simulink model "s_c856m4k_cd"  (R2016b)
(part 2 of 60)

      mask init:
      | pipeline_init(gcb,'latency',latency);
      settings: AttributesFormatString=Latency = %<latency>
      mask Display:
      | port_label('input', 1, 'd');
      | port_label('output', 1, 'q');
      | disp(['Z^-', num2str(latency)]);
  pipeline78 : Subsystem  AncestorBlock=casper_library_delays/pipeline  mask(pipeline){latency=2}
      mask help:
      | An explicitly laid-out delay line to avoid mapping to SRL16s
      | for use in pipelining to help achieve timing closure.
      mask init:
      | pipeline_init(gcb,'latency',latency);
      settings: AttributesFormatString=Latency = %<latency>
      mask Display:
      | port_label('input', 1, 'd');
      | port_label('output', 1, 'q');
      | disp(['Z^-', num2str(latency)]);
  pipeline8 : Subsystem  AncestorBlock=casper_library_delays/pipeline  mask(pipeline){latency=2}
      mask help:
      | An explicitly laid-out delay line to avoid mapping to SRL16s
      | for use in pipelining to help achieve timing closure.
      mask init:
      | pipeline_init(gcb,'latency',latency);
      settings: AttributesFormatString=Latency = %<latency>
      mask Display:
      | port_label('input', 1, 'd');
      | port_label('output', 1, 'q');
      | disp(['Z^-', num2str(latency)]);
  pipeline84 : Subsystem  AncestorBlock=casper_library_delays/pipeline  mask(pipeline){latency=2}
      mask help:
      | An explicitly laid-out delay line to avoid mapping to SRL16s
      | for use in pipelining to help achieve timing closure.
      mask init:
      | pipeline_init(gcb,'latency',latency);
      settings: AttributesFormatString=Latency = %<latency>
      mask Display:
      | port_label('input', 1, 'd');
      | port_label('output', 1, 'q');
      | disp(['Z^-', num2str(latency)]);
  pipeline88 : Subsystem  AncestorBlock=casper_library_delays/pipeline  mask(pipeline){latency=1}
      mask help:
      | An explicitly laid-out delay line to avoid mapping to SRL16s
      | for use in pipelining to help achieve timing closure.
      mask init:
      | pipeline_init(gcb,'latency',latency);
      settings: AttributesFormatString=Latency = %<latency>
      mask Display:
      | port_label('input', 1, 'd');
      | port_label('output', 1, 'q');
      | disp(['Z^-', num2str(latency)]);
  pipeline9 : Subsystem  AncestorBlock=casper_library_delays/pipeline  mask(pipeline){latency=2}
      mask help:
      | An explicitly laid-out delay line to avoid mapping to SRL16s
      | for use in pipelining to help achieve timing closure.
      mask init:
      | pipeline_init(gcb,'latency',latency);
      settings: AttributesFormatString=Latency = %<latency>
      mask Display:
      | port_label('input', 1, 'd');
      | port_label('output', 1, 'q');
      | disp(['Z^-', num2str(latency)]);
  pipeline96 : Subsystem  AncestorBlock=casper_library_delays/pipeline  mask(pipeline){latency=2}
      mask help:
      | An explicitly laid-out delay line to avoid mapping to SRL16s
      | for use in pipelining to help achieve timing closure.
      mask init:
      | pipeline_init(gcb,'latency',latency);
      settings: AttributesFormatString=Latency = %<latency>
      mask Display:
      | port_label('input', 1, 'd');
      | port_label('output', 1, 'q');
      | disp(['Z^-', num2str(latency)]);
  pipeline97 : Subsystem  AncestorBlock=casper_library_delays/pipeline  mask(pipeline){latency=2}
      mask help:
      | An explicitly laid-out delay line to avoid mapping to SRL16s
      | for use in pipelining to help achieve timing closure.
      mask init:
      | pipeline_init(gcb,'latency',latency);
      settings: AttributesFormatString=Latency = %<latency>
      mask Display:
      | port_label('input', 1, 'd');
      | port_label('output', 1, 'q');
      | disp(['Z^-', num2str(latency)]);
  pipeline98 : Subsystem  AncestorBlock=casper_library_delays/pipeline  mask(pipeline){latency=2}
      mask help:
      | An explicitly laid-out delay line to avoid mapping to SRL16s
      | for use in pipelining to help achieve timing closure.
      mask init:
      | pipeline_init(gcb,'latency',latency);
      settings: AttributesFormatString=Latency = %<latency>
      mask Display:
      | port_label('input', 1, 'd');
      | port_label('output', 1, 'q');
      | disp(['Z^-', num2str(latency)]);
  pipeline99 : Subsystem  AncestorBlock=casper_library_delays/pipeline  mask(pipeline){latency=2}
      mask help:
      | An explicitly laid-out delay line to avoid mapping to SRL16s
      | for use in pipelining to help achieve timing closure.
      mask init:
      | pipeline_init(gcb,'latency',latency);
      settings: AttributesFormatString=Latency = %<latency>
      mask Display:
      | port_label('input', 1, 'd');
      | port_label('output', 1, 'q');
      | disp(['Z^-', num2str(latency)]);
  pkt_cnt0 : Subsystem
  rx_dest_ip : Subsystem  Tag=xps:sw_reg  AncestorBlock=xps_library/software register  mask(swreg){io_dir=To Processor, io_delay=0, sample_period=1, names=reg, bitwidths=32, bin_pts=0, arith_types=0, sim_port=off, show_format=on}
      mask prompts: io_dir "I/O direction"; io_delay "I/O delay"; sample_period "Sample period"; names "Bitfield names [msb...lsb]"; bitwidths "Bitfield widths"; bin_pts "Bitfield binary pts"; arith_types "Bitfield types, ufix=0, fix=1, bool=2"; sim_port "Provide sim input/output?"; show_format "Print format string?"
      mask help: A 32-bit software-accessible register. Can be divided into bitfields of varying widths and types using the fields in the block mask.
      mask init:
      | swreg_init(gcb)
      settings: AttributesFormatString=1output:uf32.0 = 32 bits
      mask TypeOptions io_dir: To Processor | From Processor
      mask Callback io_dir:
      | mask_enables = get_param(gcb, 'MaskEnables');
      | mask_names = get_param(gcb, 'MaskNames');
      | if strcmp(get_param(gcb, 'io_dir'), 'To Processor'),
      |     mask_enables{ismember(mask_names, 'sample_period')} = 'off';
      | else
      |     mask_enables{ismember(mask_names, 'sample_period')} = 'on';
      | end
      | set_param(gcb, 'MaskEnables', mask_enables);
  rx_dest_port : Subsystem  Tag=xps:sw_reg  AncestorBlock=xps_library/software register  mask(swreg){io_dir=To Processor, io_delay=0, sample_period=1, names=reg, bitwidths=16, bin_pts=0, arith_types=0, sim_port=off, show_format=on}
      mask prompts: io_dir "I/O direction"; io_delay "I/O delay"; sample_period "Sample period"; names "Bitfield names [msb...lsb]"; bitwidths "Bitfield widths"; bin_pts "Bitfield binary pts"; arith_types "Bitfield types, ufix=0, fix=1, bool=2"; sim_port "Provide sim input/output?"; show_format "Print format string?"
      mask help: A 32-bit software-accessible register. Can be divided into bitfields of varying widths and types using the fields in the block mask.
      mask init:
      | swreg_init(gcb)
      settings: AttributesFormatString=1output:uf16.0 = 16 bits
      mask TypeOptions io_dir: To Processor | From Processor
      mask Callback io_dir:
      | mask_enables = get_param(gcb, 'MaskEnables');
      | mask_names = get_param(gcb, 'MaskNames');
      | if strcmp(get_param(gcb, 'io_dir'), 'To Processor'),
      |     mask_enables{ismember(mask_names, 'sample_period')} = 'off';
      | else
      |     mask_enables{ismember(mask_names, 'sample_period')} = 'on';
      | end
      | set_param(gcb, 'MaskEnables', mask_enables);
  rx_integrity_check0 : Subsystem
  rx_pkt_cnt_bad : Subsystem  Tag=xps:sw_reg  AncestorBlock=xps_library/software register  mask(swreg){io_dir=To Processor, io_delay=0, sample_period=1, names=reg, bitwidths=32, bin_pts=0, arith_types=0, sim_port=off, show_format=on}
      mask prompts: io_dir "I/O direction"; io_delay "I/O delay"; sample_period "Sample period"; names "Bitfield names [msb...lsb]"; bitwidths "Bitfield widths"; bin_pts "Bitfield binary pts"; arith_types "Bitfield types, ufix=0, fix=1, bool=2"; sim_port "Provide sim input/output?"; show_format "Print format string?"
      mask help: A 32-bit software-accessible register. Can be divided into bitfields of varying widths and types using the fields in the block mask.
      mask init:
      | swreg_init(gcb)
      settings: AttributesFormatString=1output:uf32.0 = 32 bits
      mask TypeOptions io_dir: To Processor | From Processor
      mask Callback io_dir:
      | mask_enables = get_param(gcb, 'MaskEnables');
      | mask_names = get_param(gcb, 'MaskNames');
      | if strcmp(get_param(gcb, 'io_dir'), 'To Processor'),
      |     mask_enables{ismember(mask_names, 'sample_period')} = 'off';
      | else
      |     mask_enables{ismember(mask_names, 'sample_period')} = 'on';
      | end
      | set_param(gcb, 'MaskEnables', mask_enables);
  rx_pkt_cnt_ok : Subsystem  Tag=xps:sw_reg  AncestorBlock=xps_library/software register  mask(swreg){io_dir=To Processor, io_delay=0, sample_period=1, names=reg, bitwidths=32, bin_pts=0, arith_types=0, sim_port=off, show_format=on}
      mask prompts: io_dir "I/O direction"; io_delay "I/O delay"; sample_period "Sample period"; names "Bitfield names [msb...lsb]"; bitwidths "Bitfield widths"; bin_pts "Bitfield binary pts"; arith_types "Bitfield types, ufix=0, fix=1, bool=2"; sim_port "Provide sim input/output?"; show_format "Print format string?"
      mask help: A 32-bit software-accessible register. Can be divided into bitfields of varying widths and types using the fields in the block mask.
      mask init:
      | swreg_init(gcb)
      settings: AttributesFormatString=1output:uf32.0 = 32 bits
      mask TypeOptions io_dir: To Processor | From Processor
      mask Callback io_dir:
      | mask_enables = get_param(gcb, 'MaskEnables');
      | mask_names = get_param(gcb, 'MaskNames');
      | if strcmp(get_param(gcb, 'io_dir'), 'To Processor'),
      |     mask_enables{ismember(mask_names, 'sample_period')} = 'off';
      | else
      |     mask_enables{ismember(mask_names, 'sample_period')} = 'on';
      | end
      | set_param(gcb, 'MaskEnables', mask_enables);
  rx_src_ip : Subsystem  Tag=xps:sw_reg  AncestorBlock=xps_library/software register  mask(swreg){io_dir=To Processor, io_delay=0, sample_period=1, names=reg, bitwidths=32, bin_pts=0, arith_types=0, sim_port=off, show_format=on}
      mask prompts: io_dir "I/O direction"; io_delay "I/O delay"; sample_period "Sample period"; names "Bitfield names [msb...lsb]"; bitwidths "Bitfield widths"; bin_pts "Bitfield binary pts"; arith_types "Bitfield types, ufix=0, fix=1, bool=2"; sim_port "Provide sim input/output?"; show_format "Print format string?"
      mask help: A 32-bit software-accessible register. Can be divided into bitfields of varying widths and types using the fields in the block mask.
      mask init:
      | swreg_init(gcb)
      settings: AttributesFormatString=1output:uf32.0 = 32 bits
      mask TypeOptions io_dir: To Processor | From Processor
      mask Callback io_dir:
      | mask_enables = get_param(gcb, 'MaskEnables');
      | mask_names = get_param(gcb, 'MaskNames');
      | if strcmp(get_param(gcb, 'io_dir'), 'To Processor'),
      |     mask_enables{ismember(mask_names, 'sample_period')} = 'off';
      | else
      |     mask_enables{ismember(mask_names, 'sample_period')} = 'on';
      | end
      | set_param(gcb, 'MaskEnables', mask_enables);
  rx_src_port : Subsystem  Tag=xps:sw_reg  AncestorBlock=xps_library/software register  mask(swreg){io_dir=To Processor, io_delay=0, sample_period=1, names=reg, bitwidths=16, bin_pts=0, arith_types=0, sim_port=off, show_format=on}
      mask prompts: io_dir "I/O direction"; io_delay "I/O delay"; sample_period "Sample period"; names "Bitfield names [msb...lsb]"; bitwidths "Bitfield widths"; bin_pts "Bitfield binary pts"; arith_types "Bitfield types, ufix=0, fix=1, bool=2"; sim_port "Provide sim input/output?"; show_format "Print format string?"
      mask help: A 32-bit software-accessible register. Can be divided into bitfields of varying widths and types using the fields in the block mask.
      mask init:
      | swreg_init(gcb)
      settings: AttributesFormatString=1output:uf16.0 = 16 bits
      mask TypeOptions io_dir: To Processor | From Processor
      mask Callback io_dir:
      | mask_enables = get_param(gcb, 'MaskEnables');
      | mask_names = get_param(gcb, 'MaskNames');
      | if strcmp(get_param(gcb, 'io_dir'), 'To Processor'),
      |     mask_enables{ismember(mask_names, 'sample_period')} = 'off';
      | else
      |     mask_enables{ismember(mask_names, 'sample_period')} = 'on';
      | end
      | set_param(gcb, 'MaskEnables', mask_enables);
  rx_status : Subsystem  Tag=xps:sw_reg  AncestorBlock=xps_library/software_register  mask(swreg){io_dir=To Processor, io_delay=0, sample_period=1, names=[badframe overrun valid eof], bitwidths=8, bin_pts=0, arith_types=0, sim_port=off, show_format=on}
      mask prompts: io_dir "I/O direction"; io_delay "I/O delay"; sample_period "Sample period"; names "Bitfield names [msb...lsb]"; bitwidths "Bitfield widths"; bin_pts "Bitfield binary pts"; arith_types "Bitfield types, ufix=0, fix=1, bool=2"; sim_port "Provide sim input/output?"; show_format "Print format string?"
      mask help: A 32-bit software-accessible register. Can be divided into bitfields of varying widths and types using the fields in the block mask.
      mask init:
      | swreg_init(gcb)
      settings: AttributesFormatString=4 outputs:uf8.0,uf8.0,uf8.0,uf8.0 = 32 bits
      mask TypeOptions io_dir: To Processor | From Processor
      mask Callback io_dir:
      | mask_enables = get_param(gcb, 'MaskEnables');
      | mask_names = get_param(gcb, 'MaskNames');
      | if strcmp(get_param(gcb, 'io_dir'), 'To Processor'),
      |     mask_enables{ismember(mask_names, 'sample_period')} = 'off';
      | else
      |     mask_enables{ismember(mask_names, 'sample_period')} = 'on';
      | end
      | set_param(gcb, 'MaskEnables', mask_enables);
      mask DialogControl ParameterTabVar0 Prompt: Setup
  rx_wrd_cnt_bad : Subsystem  Tag=xps:sw_reg  AncestorBlock=xps_library/software register  mask(swreg){io_dir=To Processor, io_delay=0, sample_period=1, names=reg, bitwidths=32, bin_pts=0, arith_types=0, sim_port=off, show_format=on}
      mask prompts: io_dir "I/O direction"; io_delay "I/O delay"; sample_period "Sample period"; names "Bitfield names [msb...lsb]"; bitwidths "Bitfield widths"; bin_pts "Bitfield binary pts"; arith_types "Bitfield types, ufix=0, fix=1, bool=2"; sim_port "Provide sim input/output?"; show_format "Print format string?"
      mask help: A 32-bit software-accessible register. Can be divided into bitfields of varying widths and types using the fields in the block mask.
      mask init:
      | swreg_init(gcb)
      settings: AttributesFormatString=1output:uf32.0 = 32 bits
      mask TypeOptions io_dir: To Processor | From Processor
      mask Callback io_dir:
      | mask_enables = get_param(gcb, 'MaskEnables');
      | mask_names = get_param(gcb, 'MaskNames');
      | if strcmp(get_param(gcb, 'io_dir'), 'To Processor'),
      |     mask_enables{ismember(mask_names, 'sample_period')} = 'off';
      | else
      |     mask_enables{ismember(mask_names, 'sample_period')} = 'on';
      | end
      | set_param(gcb, 'MaskEnables', mask_enables);
  rx_wrd_cnt_missing : Subsystem  Tag=xps:sw_reg  AncestorBlock=xps_library/software register  mask(swreg){io_dir=To Processor, io_delay=0, sample_period=1, names=reg, bitwidths=32, bin_pts=0, arith_types=0, sim_port=off, show_format=on}
      mask prompts: io_dir "I/O direction"; io_delay "I/O delay"; sample_period "Sample period"; names "Bitfield names [msb...lsb]"; bitwidths "Bitfield widths"; bin_pts "Bitfield binary pts"; arith_types "Bitfield types, ufix=0, fix=1, bool=2"; sim_port "Provide sim input/output?"; show_format "Print format string?"
      mask help: A 32-bit software-accessible register. Can be divided into bitfields of varying widths and types using the fields in the block mask.
      mask init:
      | swreg_init(gcb)
      settings: AttributesFormatString=1output:uf32.0 = 32 bits
      mask TypeOptions io_dir: To Processor | From Processor
      mask Callback io_dir:
      | mask_enables = get_param(gcb, 'MaskEnables');
      | mask_names = get_param(gcb, 'MaskNames');
      | if strcmp(get_param(gcb, 'io_dir'), 'To Processor'),
      |     mask_enables{ismember(mask_names, 'sample_period')} = 'off';
      | else
      |     mask_enables{ismember(mask_names, 'sample_period')} = 'on';
      | end
      | set_param(gcb, 'MaskEnables', mask_enables);
  snap_adc0 : Subsystem  Tag=casper:bitsnap  AncestorBlock=casper_library_scopes/bitfield snapshot  mask(bitsnap){io_names=[d0 d1 d2 d3 d4 d5 d6 d7 p1_d0 p1_d1 p1_d2 p1_d3 p1_d4_u8], io_widths=[10 10 10 10 10 10 10 10 10 10 10 10 8], io_bps=[9 9 9 9 9 9 9 9 9 9 9 9 0], io_types=[1 1 1 1 1 1 1 1 1 1 1 1 0], snap_storage=bram, snap_dram_dimm=2, snap_dram_clock=250, snap_nsamples=11, snap_data_width=128, snap_offset=on, snap_circap=off, snap_value=off, snap_use_dsp48=off, snap_delay=0, extra_names=[c d], extra_widths=[30 2], extra_bps=[0 0], extra_types=[0 0]}
      mask prompts: io_names "Names [msb...lsb]"; io_widths "Widths [msb...lsb]"; io_bps "Binary pts [msb...lsb]"; io_types "Data types [msb...lsb], ufix=0, fix=1, bool=2"; snap_storage "Storage medium"; snap_dram_dimm "DRAM dimm"; snap_dram_clock "DRAM clock rate"; snap_nsamples "Number of Samples (2^?)"; snap_data_width "Data width"; snap_offset "Start delay support"; snap_circap "Circular capture support"; snap_value "Extra value capture support"; snap_use_dsp48 "Use DSP48s to implement counters"; snap_delay "Pre-snapshot delay"; extra_names "Names [msb...lsb]"; extra_widths "Widths [msb...lsb]"; extra_bps "Binary pts [msb...lsb]"; extra_types "Data types [msb...lsb], ufix=0, fix=1, bool=2"
      mask help:
      | A wrapped snapshot block. Allows specification of inputs to a snapblock word so the toolflow can automatically set up the scope.
      | See documentation for snapshot for explanation of parameters.
      mask init:
      | bitsnap_init(gcb);
      mask TypeOptions snap_storage: bram | dram
      mask Callback snap_storage: bitsnap_callback();
      mask TypeOptions snap_dram_dimm: 1 | 2 | 3 | 4
      mask TypeOptions snap_dram_clock: 200 | 250 | 266 | 300 | 333
      mask TypeOptions snap_data_width: 8 | 16 | 32 | 64 | 128
      mask Callback snap_value: bitsnap_callback();
  snap_adc1 : Subsystem  Tag=casper:bitsnap  AncestorBlock=casper_library_scopes/bitfield snapshot  mask(bitsnap){io_names=[p1_d4_l2 p1_d5 p1_d6 p1_d7], io_widths=[2 10 10 10], io_bps=[0 9 9 9], io_types=[0 1 1 1], snap_storage=bram, snap_dram_dimm=2, snap_dram_clock=250, snap_nsamples=11, snap_data_width=32, snap_offset=on, snap_circap=off, snap_value=off, snap_use_dsp48=off, snap_delay=0, extra_names=[c d], extra_widths=[30 2], extra_bps=[0 0], extra_types=[0 0]}
      mask prompts: io_names "Names [msb...lsb]"; io_widths "Widths [msb...lsb]"; io_bps "Binary pts [msb...lsb]"; io_types "Data types [msb...lsb], ufix=0, fix=1, bool=2"; snap_storage "Storage medium"; snap_dram_dimm "DRAM dimm"; snap_dram_clock "DRAM clock rate"; snap_nsamples "Number of Samples (2^?)"; snap_data_width "Data width"; snap_offset "Start delay support"; snap_circap "Circular capture support"; snap_value "Extra value capture support"; snap_use_dsp48 "Use DSP48s to implement counters"; snap_delay "Pre-snapshot delay"; extra_names "Names [msb...lsb]"; extra_widths "Widths [msb...lsb]"; extra_bps "Binary pts [msb...lsb]"; extra_types "Data types [msb...lsb], ufix=0, fix=1, bool=2"
      mask help:
      | A wrapped snapshot block. Allows specification of inputs to a snapblock word so the toolflow can automatically set up the scope.
      | See documentation for snapshot for explanation of parameters.
      mask init:
      | bitsnap_init(gcb);
      mask TypeOptions snap_storage: bram | dram
      mask Callback snap_storage: bitsnap_callback();
      mask TypeOptions snap_dram_dimm: 1 | 2 | 3 | 4
      mask TypeOptions snap_dram_clock: 200 | 250 | 266 | 300 | 333
      mask TypeOptions snap_data_width: 8 | 16 | 32 | 64 | 128
      mask Callback snap_value: bitsnap_callback();
  spec_edge_count : Subsystem  Tag=xps:sw_reg  AncestorBlock=xps_library/software register  mask(swreg){io_dir=To Processor, io_delay=0, sample_period=1, names=reg, bitwidths=32, bin_pts=0, arith_types=0, sim_port=on, show_format=on}
      mask prompts: io_dir "I/O direction"; io_delay "I/O delay"; sample_period "Sample period"; names "Bitfield names [msb...lsb]"; bitwidths "Bitfield widths"; bin_pts "Bitfield binary pts"; arith_types "Bitfield types, ufix=0, fix=1, bool=2"; sim_port "Provide sim input/output?"; show_format "Print format string?"
      mask help: A 32-bit software-accessible register. Can be divided into bitfields of varying widths and types using the fields in the block mask.
      mask init:
      | swreg_init(gcb)
      settings: AttributesFormatString=1output:uf32.0 = 32 bits
      mask TypeOptions io_dir: To Processor | From Processor
      mask Callback io_dir:
      | mask_enables = get_param(gcb, 'MaskEnables');
      | mask_names = get_param(gcb, 'MaskNames');
      | if strcmp(get_param(gcb, 'io_dir'), 'To Processor'),
      |     mask_enables{ismember(mask_names, 'sample_period')} = 'off';
      | else
      |     mask_enables{ismember(mask_names, 'sample_period')} = 'on';
      | end
      | set_param(gcb, 'MaskEnables', mask_enables);
  status_barrel : Subsystem  Tag=xps:sw_reg  AncestorBlock=xps_library/software_register  mask(swreg){io_dir=To Processor, io_delay=0, sample_period=1, names=[dv_cnt eof_cnt hdrfix_cnt], bitwidths=10, bin_pts=0, arith_types=0, sim_port=off, show_format=on}
      mask prompts: io_dir "I/O direction"; io_delay "I/O delay"; sample_period "Sample period"; names "Bitfield names [msb...lsb]"; bitwidths "Bitfield widths"; bin_pts "Bitfield binary pts"; arith_types "Bitfield types, ufix=0, fix=1, bool=2"; sim_port "Provide sim input/output?"; show_format "Print format string?"
      mask help: A 32-bit software-accessible register. Can be divided into bitfields of varying widths and types using the fields in the block mask.
      mask init:
      | swreg_init(gcb)
      settings: AttributesFormatString=3 outputs:uf10.0,uf10.0,uf10.0 = 30 bits
      mask TypeOptions io_dir: To Processor | From Processor
      mask Callback io_dir:
      | mask_enables = get_param(gcb, 'MaskEnables');
      | mask_names = get_param(gcb, 'MaskNames');
      | if strcmp(get_param(gcb, 'io_dir'), 'To Processor'),
      |     mask_enables{ismember(mask_names, 'sample_period')} = 'off';
      | else
      |     mask_enables{ismember(mask_names, 'sample_period')} = 'on';
      | end
      | set_param(gcb, 'MaskEnables', mask_enables);
      mask DialogControl ParameterTabVar0 Prompt: Setup
  status_reo0 : Subsystem  Tag=xps:sw_reg  AncestorBlock=xps_library/software_register  mask(swreg){io_dir=To Processor, io_delay=0, sample_period=1, names=[err_disc err_relock pkt_cnt], bitwidths=10, bin_pts=0, arith_types=0, sim_port=off, show_format=on}
      mask prompts: io_dir "I/O direction"; io_delay "I/O delay"; sample_period "Sample period"; names "Bitfield names [msb...lsb]"; bitwidths "Bitfield widths"; bin_pts "Bitfield binary pts"; arith_types "Bitfield types, ufix=0, fix=1, bool=2"; sim_port "Provide sim input/output?"; show_format "Print format string?"
      mask help: A 32-bit software-accessible register. Can be divided into bitfields of varying widths and types using the fields in the block mask.
      mask init:
      | swreg_init(gcb)
      settings: AttributesFormatString=3 outputs:uf10.0,uf10.0,uf10.0 = 30 bits
      mask TypeOptions io_dir: To Processor | From Processor
      mask Callback io_dir:
      | mask_enables = get_param(gcb, 'MaskEnables');
      | mask_names = get_param(gcb, 'MaskNames');
      | if strcmp(get_param(gcb, 'io_dir'), 'To Processor'),
      |     mask_enables{ismember(mask_names, 'sample_period')} = 'off';
      | else
      |     mask_enables{ismember(mask_names, 'sample_period')} = 'on';
      | end
      | set_param(gcb, 'MaskEnables', mask_enables);
  status_reo1 : Subsystem  Tag=xps:sw_reg  AncestorBlock=xps_library/software_register  mask(swreg){io_dir=To Processor, io_delay=0, sample_period=1, names=[err_pkttime err_timestep err_recv err_of], bitwidths=8, bin_pts=0, arith_types=0, sim_port=off, show_format=on}
      mask prompts: io_dir "I/O direction"; io_delay "I/O delay"; sample_period "Sample period"; names "Bitfield names [msb...lsb]"; bitwidths "Bitfield widths"; bin_pts "Bitfield binary pts"; arith_types "Bitfield types, ufix=0, fix=1, bool=2"; sim_port "Provide sim input/output?"; show_format "Print format string?"
      mask help: A 32-bit software-accessible register. Can be divided into bitfields of varying widths and types using the fields in the block mask.
      mask init:
      | swreg_init(gcb)
      settings: AttributesFormatString=4 outputs:uf8.0,uf8.0,uf8.0,uf8.0 = 32 bits
      mask TypeOptions io_dir: To Processor | From Processor
      mask Callback io_dir:
      | mask_enables = get_param(gcb, 'MaskEnables');
      | mask_names = get_param(gcb, 'MaskNames');
      | if strcmp(get_param(gcb, 'io_dir'), 'To Processor'),
      |     mask_enables{ismember(mask_names, 'sample_period')} = 'off';
      | else
      |     mask_enables{ismember(mask_names, 'sample_period')} = 'on';
      | end
      | set_param(gcb, 'MaskEnables', mask_enables);
  status_spead0 : Subsystem  Tag=xps:sw_reg  AncestorBlock=xps_library/software_register  mask(swreg){io_dir=To Processor, io_delay=0, sample_period=1, names=[err_magic err_hdr err_pad err_len pkt_cnt], bitwidths=6, bin_pts=0, arith_types=0, sim_port=off, show_format=on}
      mask prompts: io_dir "I/O direction"; io_delay "I/O delay"; sample_period "Sample period"; names "Bitfield names [msb...lsb]"; bitwidths "Bitfield widths"; bin_pts "Bitfield binary pts"; arith_types "Bitfield types, ufix=0, fix=1, bool=2"; sim_port "Provide sim input/output?"; show_format "Print format string?"
      mask help: A 32-bit software-accessible register. Can be divided into bitfields of varying widths and types using the fields in the block mask.
      mask init:
      | swreg_init(gcb)
      settings: AttributesFormatString=5 outputs:uf6.0,uf6.0,uf6.0,uf6.0,uf6.0 = 30 bits
      mask TypeOptions io_dir: To Processor | From Processor
      mask Callback io_dir:
      | mask_enables = get_param(gcb, 'MaskEnables');
      | mask_names = get_param(gcb, 'MaskNames');
      | if strcmp(get_param(gcb, 'io_dir'), 'To Processor'),
      |     mask_enables{ismember(mask_names, 'sample_period')} = 'off';
      | else
      |     mask_enables{ismember(mask_names, 'sample_period')} = 'on';
      | end
      | set_param(gcb, 'MaskEnables', mask_enables);
  status_spead1 : Subsystem  Tag=xps:sw_reg  AncestorBlock=xps_library/software_register  mask(swreg){io_dir=To Processor, io_delay=0, sample_period=1, names=[err_time0 err_time1 err_time2 err_time_heap err_pkt_ooo], bitwidths=6, bin_pts=0, arith_types=0, sim_port=off, show_format=on}
      mask prompts: io_dir "I/O direction"; io_delay "I/O delay"; sample_period "Sample period"; names "Bitfield names [msb...lsb]"; bitwidths "Bitfield widths"; bin_pts "Bitfield binary pts"; arith_types "Bitfield types, ufix=0, fix=1, bool=2"; sim_port "Provide sim input/output?"; show_format "Print format string?"
      mask help: A 32-bit software-accessible register. Can be divided into bitfields of varying widths and types using the fields in the block mask.
      mask init:
      | swreg_init(gcb)
      settings: AttributesFormatString=5 outputs:uf6.0,uf6.0,uf6.0,uf6.0,uf6.0 = 30 bits
      mask TypeOptions io_dir: To Processor | From Processor
      mask Callback io_dir:
      | mask_enables = get_param(gcb, 'MaskEnables');
      | mask_names = get_param(gcb, 'MaskNames');
      | if strcmp(get_param(gcb, 'io_dir'), 'To Processor'),
      |     mask_enables{ismember(mask_names, 'sample_period')} = 'off';
      | else
      |     mask_enables{ismember(mask_names, 'sample_period')} = 'on';
      | end
      | set_param(gcb, 'MaskEnables', mask_enables);
  sync_gen : Subsystem  mask{zerolsbs=((15 + 1) + 8)}
      mask prompts: zerolsbs "No. LSBs to be zero:"
  tl_cd0 : Subsystem  mask(timed_latch){n_bits_time=48-fft_stages, n_bits_quantization=fft_stages, n_bits_counters=4}
      mask prompts: n_bits_time "Number bits in time to compare"; n_bits_quantization "Time offset from lsb"; n_bits_counters "Bits in status counters"
      mask help:
      | Latches load_value when armed and current_time matches requested time.
      | current_time should be in ADC samples.
      mask init:
      | set_param([gcb,'/status'], 'bitwidths', mat2str([1, repmat(n_bits_counters, 1, 2)]));
      mask Help:
      | When armed, will latch new value when current time matches the time
      | specified. The input time should be in samples and mask settings allow
      | a portion of this to be compared to cater for quantization. Arm and latch
      | counts allow the current state, pending and missed latch events to be
      | determined.
  tl_cd1 : Subsystem  mask(timed_latch){n_bits_time=48-fft_stages, n_bits_quantization=fft_stages, n_bits_counters=4}
      mask prompts: n_bits_time "Number bits in time to compare"; n_bits_quantization "Time offset from lsb"; n_bits_counters "Bits in status counters"
      mask help:
      | Latches load_value when armed and current_time matches requested time.
      | current_time should be in ADC samples.
      mask init:
      | set_param([gcb,'/status'], 'bitwidths', mat2str([1, repmat(n_bits_counters, 1, 2)]));
      mask Help:
      | When armed, will latch new value when current time matches the time
      | specified. The input time should be in samples and mask settings allow
      | a portion of this to be compared to cater for quantization. Arm and latch
      | counts allow the current state, pending and missed latch events to be
      | determined.
  trig_time_lsw : Subsystem  Tag=xps:sw_reg  AncestorBlock=xps_library/software register  mask(swreg){io_dir=From Processor, io_delay=0, sample_period=1, names=lsw, bitwidths=32, bin_pts=0, arith_types=0, sim_port=off, show_format=on}
      mask prompts: io_dir "I/O direction"; io_delay "I/O delay"; sample_period "Sample period"; names "Bitfield names [msb...lsb]"; bitwidths "Bitfield widths"; bin_pts "Bitfield binary pts"; arith_types "Bitfield types, ufix=0, fix=1, bool=2"; sim_port "Provide sim input/output?"; show_format "Print format string?"
      mask help: A 32-bit software-accessible register. Can be divided into bitfields of varying widths and types using the fields in the block mask.
      mask init:
      | swreg_init(gcb)
      settings: AttributesFormatString=1input:uf32.0 = 32 bits
      mask TypeOptions io_dir: To Processor | From Processor
      mask Callback io_dir:
      | mask_enables = get_param(gcb, 'MaskEnables');
      | mask_names = get_param(gcb, 'MaskNames');
      | if strcmp(get_param(gcb, 'io_dir'), 'To Processor'),
      |     mask_enables{ismember(mask_names, 'sample_period')} = 'off';
      | else
      |     mask_enables{ismember(mask_names, 'sample_period')} = 'on';
      | end
      | set_param(gcb, 'MaskEnables', mask_enables);
  trig_time_msw : Subsystem  Tag=xps:sw_reg  AncestorBlock=xps_library/software register  mask(swreg){io_dir=From Processor, io_delay=0, sample_period=1, names=msw, bitwidths=16, bin_pts=0, arith_types=0, sim_port=off, show_format=on}
      mask prompts: io_dir "I/O direction"; io_delay "I/O delay"; sample_period "Sample period"; names "Bitfield names [msb...lsb]"; bitwidths "Bitfield widths"; bin_pts "Bitfield binary pts"; arith_types "Bitfield types, ufix=0, fix=1, bool=2"; sim_port "Provide sim input/output?"; show_format "Print format string?"
      mask help: A 32-bit software-accessible register. Can be divided into bitfields of varying widths and types using the fields in the block mask.
      mask init:
      | swreg_init(gcb)
      settings: AttributesFormatString=1input:uf16.0 = 16 bits
      mask TypeOptions io_dir: To Processor | From Processor
      mask Callback io_dir:
      | mask_enables = get_param(gcb, 'MaskEnables');
      | mask_names = get_param(gcb, 'MaskNames');
      | if strcmp(get_param(gcb, 'io_dir'), 'To Processor'),
      |     mask_enables{ismember(mask_names, 'sample_period')} = 'off';
      | else
      |     mask_enables{ismember(mask_names, 'sample_period')} = 'on';
      | end
      | set_param(gcb, 'MaskEnables', mask_enables);
  tx_metadata : Subsystem  Tag=xps:sw_reg  AncestorBlock=xps_library/software register  mask(swreg){io_dir=From Processor, io_delay=0, sample_period=1, names=[porttx board_id], bitwidths=16, bin_pts=0, arith_types=0, sim_port=off, show_format=on}
      mask prompts: io_dir "I/O direction"; io_delay "I/O delay"; sample_period "Sample period"; names "Bitfield names [msb...lsb]"; bitwidths "Bitfield widths"; bin_pts "Bitfield binary pts"; arith_types "Bitfield types, ufix=0, fix=1, bool=2"; sim_port "Provide sim input/output?"; show_format "Print format string?"
      mask help: A 32-bit software-accessible register. Can be divided into bitfields of varying widths and types using the fields in the block mask.
      mask init:
      | swreg_init(gcb)
      settings: AttributesFormatString=2 inputs:uf16.0,uf16.0 = 32 bits
      mask TypeOptions io_dir: To Processor | From Processor
      mask Callback io_dir:
      | mask_enables = get_param(gcb, 'MaskEnables');
      | mask_names = get_param(gcb, 'MaskNames');
      | if strcmp(get_param(gcb, 'io_dir'), 'To Processor'),
      |     mask_enables{ismember(mask_names, 'sample_period')} = 'off';
      | else
      |     mask_enables{ismember(mask_names, 'sample_period')} = 'on';
      | end
      | set_param(gcb, 'MaskEnables', mask_enables);
  unpack_and_reorder : Subsystem
  unpack_control : Subsystem  Tag=xps:sw_reg  AncestorBlock=xps_library/software_register  mask(swreg){io_dir=From Processor, io_delay=0, sample_period=1, names=[cnt_rst], bitwidths=1, bin_pts=0, arith_types=2, sim_port=off, show_format=on}
      mask prompts: io_dir "I/O direction"; io_delay "I/O delay"; sample_period "Sample period"; names "Bitfield names [msb...lsb]"; bitwidths "Bitfield widths"; bin_pts "Bitfield binary pts"; arith_types "Bitfield types, ufix=0, fix=1, bool=2"; sim_port "Provide sim input/output?"; show_format "Print format string?"
      mask help: A 32-bit software-accessible register. Can be divided into bitfields of varying widths and types using the fields in the block mask.
      mask init:
      | swreg_init(gcb)
      settings: AttributesFormatString=1input:b = 1 bits
      mask TypeOptions io_dir: To Processor | From Processor
      mask Callback io_dir:
      | mask_enables = get_param(gcb, 'MaskEnables');
      | mask_names = get_param(gcb, 'MaskNames');
      | if strcmp(get_param(gcb, 'io_dir'), 'To Processor'),
      |     mask_enables{ismember(mask_names, 'sample_period')} = 'off';
      | else
      |     mask_enables{ismember(mask_names, 'sample_period')} = 'on';
      | end
      | set_param(gcb, 'MaskEnables', mask_enables);
      mask DialogControl ParameterTabVar0 Prompt: Setup
  xsg_core_config : Subsystem  Tag=xps:xsg  AncestorBlock=xps_library/XSG_core_config  mask(xsg core config){hw_sys=SKARAB:xc7vx690t, clk_src=sys_clk, clk_rate=238, sample_period=1, synthesis_tool=XST}
      mask prompts: hw_sys "Hardware Platform"; clk_src "User IP Clock source"; clk_rate "User IP Clock Rate (MHz)"; sample_period "Sample Period"; synthesis_tool "Synthesis Tool:"
      mask help:
      | The XSG Core Config block is used to configure the System Generator design
      | for the casper_xps toolflow. Settings here are used to configure the
      | Xilinx System Generator block parameters automatically, and control toolflow
      | script  execution. It needs to be at the top level of all designs being compiled
      | with the casper_xps toolflow.
      mask init:
      | xps_xsg_conf_mask;
      mask Help: eval('xlWeb([getenv(''MLIB_ROOT''), ''\doc\html\sys_xsg_core_config\sys_xsg_core_config.html''])')
      mask TypeOptions hw_sys: ROACH:sx95t | ROACH:lx110t | ROACH2:sx475t | SNAP:xc7k160t | KC705:xc7k325t | SKARAB:xc7vx690t
      mask Callback hw_sys: xps_xsg_conf_callback
      mask TypeOptions clk_src: sys_clk | aux_clk
      mask Callback clk_src: xps_xsg_conf_callback
      mask Callback clk_rate: xps_xsg_conf_callback
      mask TypeOptions synthesis_tool: Leonardo Spectrum | Synplify | Synplify Pro | XST
      mask Display: fprintf(['MSSGE\n', hw_sys]);
  tag scope: cnt_rst=global, sys_rst=global
  wires:
  Constant3/1 -> gbe0/8(rx_overrun_ack)
  Constant4/1 -> gbe0/7(rx_ack)
  [gbe_rst] -> pipeline99/1(d)
  [cnt_rst] -> rx_integrity_check0/1(rst)
  pkt_cnt0/1(ok_cnt) -> rx_pkt_cnt_ok/1(out_reg)
  pkt_cnt0/2(bad_cnt) -> rx_pkt_cnt_bad/1(out_reg)
  [cnt_rst] -> pkt_cnt0/1(rst)
  [forty_gbe_rx_bad] -> pkt_cnt0/4(bad)
  [forty_gbe_rx_eof] -> pkt_cnt0/3(eof)
  [forty_gbe_rx_valid] -> pkt_cnt0/2(valid), rx_integrity_check0/3(en_in)
  [forty_gbe_rx_data] -> rx_integrity_check0/2(data_in)
  unpack_and_reorder/5(recvd) -> pipeline17/1(d)
  sync_gen/2(dout) -> bus_expand6/1(bus_in)
  sync_gen/3(dvalid) -> Gateway Out39/1, impulse_gen0/6(en), impulse_gen1/6(en)
  Slice4/1 -> pipeline16/1(d)
  pipeline16/1(q) -> local_time_lsw/1(out_timestamp_lsw)
  Slice16/1 -> Convert6/1
  pipeline47/1(q) -> local_time_msw/1(out_timestamp_msw)
  Convert6/1 -> pipeline47/1(d)
  [time80_48] -> Slice16/1, Slice4/1
  Concat22/1 -> [ld_val0]
  Concat3/1 -> [ld_val1]
  bus_expand17/1(msb_out2) -> [unpack_recvd0]
  bus_expand17/2(lsb_out1) -> [unpack_recvd1]
  Slice12/1 -> [time80]
  impulse_gen0/3(dvalid) -> Gateway Out34/1, [valid80]
  impulse_gen0/1(sync_out) -> Gateway Out33/1, [sync80]
  impulse_gen0/2(dout) -> Gateway Out35/1, [d80_adc0]
  impulse_gen0/4(misco) -> [time80_48], Slice12/1
  [tvg_adc_en] -> impulse_gen0/1(tvg_en)
  impulse_gen1/1(sync_out) -> Gateway Out64/1, Terminator6/1
  impulse_gen1/2(dout) -> Gateway Out65/1, [d80_adc1]
  impulse_gen1/3(dvalid) -> Gateway Out63/1, Terminator8/1
  impulse_gen1/4(misco) -> [dig_flags]
  [tvg_adc_en] -> impulse_gen1/1(tvg_en)
  impulse0/1(in_offset) -> Slice7/1
  impulse0/2(in_amplitude) -> impulse_gen0/3(impulse_amplitude), Gateway Out16/1
  impulse1/1(in_offset) -> Slice8/1
  impulse1/2(in_amplitude) -> impulse_gen1/3(impulse_amplitude)
  sync_gen/1(sync) -> impulse_gen0/4(sync_in), impulse_gen1/4(sync_in)
  bus_expand6/1(msb_out2) -> impulse_gen0/5(din)
  bus_expand6/2(lsb_out1) -> impulse_gen1/5(din)
  sync_gen/5(misco) -> impulse_gen1/7(misci)
  sync_gen/4(time_out) -> impulse_gen0/7(misci)
  Constant31/1 -> Concat9/2
  [unpack_timestamp] -> Concat9/1
  [up_timestep_error] -> Logical15/1
  [sys_rst] -> Logical15/2
  Logical15/1 -> edge_detect17/1(in)
  edge_detect17/1(out) -> [sys_relock]
  phase0/1(in_initial) -> Reinterpret2/1
  delta_delay0/1(in_delta) -> Reinterpret1/1
  phase0/2(in_delta) -> Reinterpret3/1
  Concat9/1 -> sync_gen/1(time_in)
  [sys_relock] -> sync_gen/5(relock)
  [unpack_d160] -> sync_gen/3(din)
  Slice7/1 -> impulse_gen0/2(impulse_offset)
  Slice8/1 -> impulse_gen1/2(impulse_offset)
  Reinterpret8/1 -> Concat22/1
  Reinterpret1/1 -> Concat22/2
  Reinterpret2/1 -> Concat22/3
  Reinterpret3/1 -> Concat22/4
  phase1/1(in_initial) -> Reinterpret5/1
  delta_delay1/1(in_delta) -> Reinterpret4/1
  phase1/2(in_delta) -> Reinterpret6/1
  Reinterpret4/1 -> Concat3/2
  Reinterpret5/1 -> Concat3/3
  Reinterpret6/1 -> Concat3/4
  Reinterpret7/1 -> Concat3/1
  delay0/1(in_initial) -> Reinterpret8/1
  delay1/1(in_initial) -> Reinterpret7/1
  trig_time_msw/1(in_msw) -> pipeline28/1(d)
  trig_time_lsw/1(in_lsw) -> pipeline44/1(d)
  Concat13/1 -> Relational10/1
  pipeline28/1(q) -> Concat13/1
  pipeline44/1(q) -> Concat13/2
  [valid80] -> Counter/2
  [sync80] -> Counter/1
  Constant12/1 -> Relational7/2
  Counter/1 -> Relational7/1
  Relational10/1 -> Mux/2
  Relational7/1 -> Mux/3
  [valid80] -> Delay49/1
  Logical12/1 -> Logical14/1
  Logical14/1 -> [adc_snap_trig]
  [adc_snap_arm] -> Logical14/2
  [time80_48] -> Relational10/2
  Delay49/1 -> Logical12/2
  Mux/1 -> Logical12/1
  [adc_snap_trig_source] -> Mux/1
  iptx_base/1(in_reg) -> pipeline105/1(d)
  pipeline105/1(q) -> [tx_ip_base]
  tx_metadata/1(in_porttx) -> pipeline106/1(d)
  tx_metadata/2(in_board_id) -> pipeline107/1(d)
  pipeline106/1(q) -> [tx_port]
  pipeline107/1(q) -> [tx_board_id]
  edge_detect4/1(out) -> pipeline5/1(d)
  control/6(in_cnt_rst) -> edge_detect1/1(in)
  edge_detect1/1(out) -> pipeline14/1(d)
  control/3(in_gbe_rst) -> pipeline6/1(d)
  control/1(in_sys_rst) -> pipeline3/1(d)
  pipeline3/1(q) -> [sys_rst]
  pipeline5/1(q) -> [clr_status]
  pipeline6/1(q) -> [gbe_rst]
  pipeline7/1(q) -> [gbe_txen]
  pipeline14/1(q) -> [cnt_rst]
  control/5(in_tvg_adc) -> pipeline13/1(d)
  edge_detect2/1(out) -> pipeline38/1(d)
  pipeline38/1(q) -> [gbe_cnt_rst]
  control/7(in_gbe_cnt_rst) -> edge_detect2/1(in)
  control/4(in_gbe_txen) -> pipeline7/1(d)
  control/2(in_status_clr) -> edge_detect4/1(in)
  pipeline43/1(q) -> [adc_snap_arm]
  control/8(in_adc_snap_arm) -> pipeline43/1(d)
  control/9(in_adc_snap_trig_select) -> pipeline39/1(d)
  pipeline39/1(q) -> [adc_snap_trig_source]
  [ld_val0] -> Gateway Out175/1, pipeline23/1(d)
  [clr_status] -> pipeline22/1(d), pipeline34/1(d)
  tl_cd0/6(time) -> Terminator16/1
  tl_cd0/3(sync_out) -> cd_compensation0/1(sync_in)
  tl_cd0/4(dout) -> cd_compensation0/2(din)
  tl_cd0/5(dvalid) -> cd_compensation0/3(en)
  tl_cd0/1(value) -> cd_compensation0/4(delay_val)
  tl_cd0/2(enable) -> cd_compensation0/5(load_val)
  Constant6/1 -> Concat15/2
  Concat15/1 -> pipeline33/1(d), pipeline21/1(d)
  [time80] -> Concat15/1
  [d80_adc0] -> pipeline25/1(d)
  pipeline22/1(q) -> tl_cd0/1(rst)
  pipeline21/1(q) -> tl_cd0/2(current_time)
  pipeline23/1(q) -> tl_cd0/3(load_value)
  pipeline24/1(q) -> tl_cd0/4(sync_in)
  pipeline25/1(q) -> tl_cd0/5(din)
  pipeline26/1(q) -> tl_cd0/6(en)
  [sync80] -> pipeline24/1(d), pipeline36/1(d)
  [valid80] -> pipeline26/1(d), pipeline40/1(d)
  tl_cd1/6(time) -> Terminator7/1
  tl_cd1/3(sync_out) -> cd_compensation1/1(sync_in)
  tl_cd1/4(dout) -> cd_compensation1/2(din)
  tl_cd1/5(dvalid) -> cd_compensation1/3(en)
  tl_cd1/1(value) -> cd_compensation1/4(delay_val)
  tl_cd1/2(enable) -> cd_compensation1/5(load_val)
  pipeline40/1(q) -> tl_cd1/6(en)
  pipeline37/1(q) -> tl_cd1/5(din)
  pipeline36/1(q) -> tl_cd1/4(sync_in)
  pipeline35/1(q) -> tl_cd1/3(load_value)
  pipeline33/1(q) -> tl_cd1/2(current_time)
  pipeline34/1(q) -> tl_cd1/1(rst)
  [ld_val1] -> Gateway Out70/1, pipeline35/1(d)
  [d80_adc1] -> pipeline37/1(d)
  [gbe_cnt_rst] -> pipeline31/1(d)
  pipeline31/1(q) -> gbe0/9(debug_rst)
  gbe0/13(rx_dest_ip) -> pipeline115/1(d)
  gbe0/14(rx_dest_port) -> pipeline116/1(d)
  [rx_dest_ip] -> pipeline/1(d)
  pipeline/1(q) -> rx_dest_ip/1(out_reg)
  [rx_dest_port] -> pipeline18/1(d)
  pipeline18/1(q) -> rx_dest_port/1(out_reg)
  gbe0/1(led_up) -> pipeline100/1(d)
  [forty_gbe_led_up] -> pipeline19/1(d)
  gbe0/2(led_rx) -> pipeline101/1(d)
  [forty_gbe_led_rx] -> pipeline20/1(d)
  gbe0/3(led_tx) -> pipeline102/1(d)
  [forty_gbe_led_tx] -> pipeline51/1(d)
  gbe0/4(tx_afull) -> pipeline103/1(d)
  [forty_gbe_tx_full] -> pipeline52/1(d)
  gbe0/5(tx_overflow) -> pipeline104/1(d)
  [forty_gbe_tx_of] -> pipeline53/1(d)
  gbe0/12(rx_overrun) -> pipeline114/1(d)
  [forty_gbe_rx_overrun] -> pipeline54/1(d)
  pipeline19/1(q) -> forty_gbe_status/1(out_led_up)
  pipeline20/1(q) -> forty_gbe_status/2(out_led_rx)
  pipeline51/1(q) -> forty_gbe_status/3(out_led_tx)
  pipeline52/1(q) -> forty_gbe_status/4(out_tx_full)
  pipeline53/1(q) -> forty_gbe_status/5(out_tx_of)
  pipeline54/1(q) -> forty_gbe_status/6(out_rx_of)
  gbe0/8(rx_source_ip) -> pipeline110/1(d)
  gbe0/9(rx_source_port) -> pipeline111/1(d)
  pipeline55/1(q) -> rx_src_ip/1(out_reg)
  pipeline56/1(q) -> rx_src_port/1(out_reg)
  [forty_gbe_rx_src_port] -> pipeline56/1(d)
  [forty_gbe_rx_src_ip] -> pipeline55/1(d)
  gbe0/6(rx_data) -> pipeline108/1(d)
  gbe0/7(rx_valid) -> pipeline109/1(d)
  gbe0/10(rx_end_of_frame) -> pipeline112/1(d)
  gbe0/11(rx_bad_frame) -> pipeline113/1(d)
  [s256_d] -> pipeline98/1(d)
  [s256_ip] -> pipeline97/1(d)
  [s256_port] -> pipeline96/1(d)
  Logical2/1 -> gbe0/6(tx_end_of_frame)
  [s256_v] -> Logical1/2
  [s256_eof] -> Logical2/2
  Delay1/1 -> Logical1/1, Logical2/1
  [s256_eof] -> Delay1/2
  pipeline96/1(q) -> gbe0/5(tx_dest_port)
  pipeline97/1(q) -> gbe0/4(tx_dest_ip)
  pipeline98/1(q) -> gbe0/2(tx_data)
  pipeline99/1(q) -> gbe0/1(rst)
  [gbe_txen] -> Delay1/1
  pipeline100/1(q) -> [forty_gbe_led_up]
  pipeline101/1(q) -> [forty_gbe_led_rx]
  pipeline102/1(q) -> [forty_gbe_led_tx]
  pipeline103/1(q) -> [forty_gbe_tx_full]
  pipeline104/1(q) -> [forty_gbe_tx_of]
  pipeline108/1(q) -> [forty_gbe_rx_data]
  pipeline110/1(q) -> [forty_gbe_rx_src_ip]
  pipeline111/1(q) -> [forty_gbe_rx_src_port]
  pipeline112/1(q) -> [forty_gbe_rx_eof]
  pipeline113/1(q) -> [forty_gbe_rx_bad]
  pipeline114/1(q) -> [forty_gbe_rx_overrun]
  pipeline115/1(q) -> [rx_dest_ip]
  pipeline116/1(q) -> [rx_dest_port]
  [forty_gbe_rx_data] -> unpack_and_reorder/1(d256)
  [forty_gbe_rx_valid] -> unpack_and_reorder/2(dv256)
  [forty_gbe_rx_eof] -> unpack_and_reorder/3(eof256)
  pipeline109/1(q) -> [forty_gbe_rx_valid]
  unpack_and_reorder/6(flags) -> Terminator9/1
  unpack_and_reorder/2(d160) -> pipeline11/1(d)
  unpack_and_reorder/3(dv) -> pipeline12/1(d)
  unpack_and_reorder/4(time) -> pipeline15/1(d)
  unpack_and_reorder/1(sync) -> pipeline10/1(d)
  Inverter1/1 -> Logical6/1
  [unpack_recvd0] -> Inverter1/1
  [unpack_dv] -> Logical6/2
  Inverter2/1 -> Logical7/1
  [unpack_recvd1] -> Inverter2/1
  [unpack_dv] -> Logical7/2
  Logical7/1 -> Logical/2
  Logical6/1 -> Logical/1
  Logical/1 -> [unpack_missing]
  pipeline10/1(q) -> [unpack_sync]
  pipeline11/1(q) -> [unpack_d160]
  pipeline12/1(q) -> [unpack_dv]
  pipeline15/1(q) -> [unpack_timestamp]
  pipeline17/1(q) -> bus_expand17/1(bus_in)
  [up_dbg_rst] -> Subsystem4/1(rst)
  [upg_sp_dv] -> Logical3/2
  [upg_sp_eof] -> Logical3/1
  [up_dbg_rst] -> Subsystem/1(debug_reset)
  [upg_sp_dv] -> Subsystem/2(dv)
  Subsystem/1(time_err0) -> status_spead1/1(out_err_time0)
  Subsystem/2(time_err1) -> status_spead1/2(out_err_time1)
  Subsystem/3(time_err2) -> status_spead1/3(out_err_time2)
  Subsystem/4(time_heapid_mismatch) -> status_spead1/4(out_err_time_heap)
  [up_dbg_rst] -> Counter23/1
  Counter23/1 -> status_reo1/4(out_err_of)
  unpack_control/1(in_cnt_rst) -> pipeline1/1(d)
  pipeline1/1(q) -> [up_dbg_rst]
  [up_dbg_rst] -> Subsystem5/1(rst)
  [upg_reo_sync] -> Subsystem1/3(sync)
  [upg_reo_time] -> Subsystem1/4(time)
  [upg_reo_recv] -> Subsystem1/5(recv)
  [upg_reo_dv] -> Subsystem1/2(dv)
  Subsystem1/1(pkt_time_err) -> status_reo1/1(out_err_pkttime)
  Subsystem1/2(timestep_err) -> status_reo1/2(out_err_timestep)
  Subsystem1/3(recv_err) -> status_reo1/3(out_err_recv)
  [up_dbg_rst] -> Subsystem1/1(debug_reset)
  Subsystem1/4(time_change) -> [reo_time_change]
  [upg_reo_disc] -> [unpack_discarding], Subsystem5/2(in0)
  [upg_reo_relock] -> Subsystem5/3(in1), [unpack_mcnt_relock]
  [reo_time_change] -> Subsystem5/4(in2)
  Logical5/1 -> Counter23/2
  [upg_of80_p1] -> Logical5/2
  [upg_of80_p0] -> Logical5/1
  [upg_sperr_magic] -> Subsystem4/2(in0)
  [upg_sperr_len] -> Subsystem4/5(in3)
  [upg_sperr_hdr] -> Subsystem4/3(in1)
  [upg_sperr_pad] -> Subsystem4/4(in2)
  Subsystem/5(packets_ooo) -> status_spead1/5(out_err_pkt_ooo)
  Constant16/1 -> tl_cd0/7(misci)
  Constant17/1 -> tl_cd1/7(misci)
  tl_cd0/7(misco) -> Terminator/1
  tl_cd1/7(misco) -> Terminator1/1
  [forty_gbe_rx_valid] -> Subsystem2/4(in2)
  [forty_gbe_rx_bad] -> Subsystem2/2(in0)
  [forty_gbe_rx_overrun] -> Subsystem2/3(in1)
  [forty_gbe_rx_eof] -> Subsystem2/5(in3)
  [up_dbg_rst] -> Subsystem2/1(rst)
  Subsystem2/4(out3) -> rx_status/4(out_eof)
  Subsystem2/2(out1) -> rx_status/2(out_overrun)
  Subsystem2/1(out0) -> rx_status/1(out_badframe)
  Subsystem2/3(out2) -> rx_status/3(out_valid)
  rx_integrity_check0/1(fail_cnt) -> rx_wrd_cnt_bad/1(out_reg)
  rx_integrity_check0/2(offset) -> rx_wrd_cnt_missing/1(out_reg)
  [up_dbg_rst] -> Subsystem3/1(rst)
  [upg_barrel_dv] -> Subsystem3/2(in0)
  [upg_barrel_eof] -> Subsystem3/3(in1)
  [upg_barrel_hdr_edit] -> Subsystem3/4(in2)
  Subsystem3/1(out0) -> status_barrel/1(out_dv_cnt)
  Subsystem3/2(out1) -> status_barrel/2(out_eof_cnt)
  Subsystem3/3(out2) -> status_barrel/3(out_hdrfix_cnt)
  Subsystem4/5(out4) -> status_spead0/5(out_pkt_cnt)
  Subsystem4/2(out1) -> status_spead0/2(out_err_hdr)
  Subsystem4/3(out2) -> status_spead0/3(out_err_pad)
  Subsystem4/1(out0) -> status_spead0/1(out_err_magic)
  Subsystem4/4(out3) -> status_spead0/4(out_err_len)
  Logical3/1 -> Subsystem4/6(in4)
  [upg_sp_eof] -> Subsystem/3(eof)
  [upg_sp_timestamp] -> Subsystem/4(timestamp48)  "sp_time"
  [upg_sp_heapid] -> Subsystem/5(heap_id)
  [upg_sp_0x3101] -> Slice/1
  Subsystem5/3(out2) -> status_reo0/3(out_pkt_cnt)
  Subsystem5/1(out0) -> status_reo0/1(out_err_disc)
  Subsystem5/2(out1) -> status_reo0/2(out_err_relock)
  Constant1/1 -> sync_gen/4(misci)
  Slice/1 -> Subsystem/6(pol_id)
  [d80_adc1] -> pipeline62/1(d)
  [d80_adc0] -> pipeline57/1(d)
  bus_expand1/1(msb_out8) -> snap_adc0/1(in_d0)
  bus_expand1/2(out7) -> snap_adc0/2(in_d1)
  bus_expand1/3(out6) -> snap_adc0/3(in_d2)
  bus_expand1/4(out5) -> snap_adc0/4(in_d3)
  bus_expand1/5(out4) -> snap_adc0/5(in_d4)
  bus_expand1/6(out3) -> snap_adc0/6(in_d5)
  bus_expand1/7(out2) -> snap_adc0/7(in_d6)
  bus_expand1/8(lsb_out1) -> snap_adc0/8(in_d7)
  bus_expand2/5(out4) -> Reinterpret/1
  pipeline57/1(q) -> bus_expand1/1(bus_in)
  Reinterpret/1 -> bus_expand3/1(bus_in)
  pipeline62/1(q) -> bus_expand2/1(bus_in)
  [valid80] -> Counter2/2, snap_adc1/5(we), snap_adc0/14(we)
  [adc_snap_trig] -> Counter1/2, snap_adc1/6(trig), snap_adc0/15(trig)
  bus_expand2/2(out7) -> snap_adc0/10(in_p1_d1)
  bus_expand2/3(out6) -> snap_adc0/11(in_p1_d2)
  bus_expand2/4(out5) -> snap_adc0/12(in_p1_d3)
  bus_expand2/1(msb_out8) -> snap_adc0/9(in_p1_d0)
  bus_expand2/6(out3) -> snap_adc1/2(in_p1_d5)
  bus_expand2/7(out2) -> snap_adc1/3(in_p1_d6)
  bus_expand2/8(lsb_out1) -> snap_adc1/4(in_p1_d7)
  bus_expand3/1(msb_out2) -> snap_adc0/13(in_p1_d4_u8)
  bus_expand3/2(lsb_out1) -> snap_adc1/1(in_p1_d4_l2)
  [d80_adc0] -> [delay_d0]
  [d80_adc1] -> [delay_d1]
  [valid80] -> [delay_dv]
  [sync80] -> [delay_sync]
  Logical1/1 -> gbe0/3(tx_valid)
  pipeline59/1(q) -> [ct_tvg_en]
  control/10(in_ct_tvg_en) -> pipeline59/1(d)
  bus_expand7/1(msb_out8) -> pipeline133/1(d)  "hmc_out9"
  bus_expand7/8(lsb_out1) -> pipeline140/1(d)  "hmc_out16"
  [cd_out_pol1] -> bus_expand8/1(bus_in), bus_expand7/1(bus_in)
  pipeline140/1(q) -> cd_out1/8(in_d07)
  pipeline139/1(q) -> cd_out1/7(in_d06)
  pipeline138/1(q) -> cd_out1/6(in_d05)
  pipeline137/1(q) -> cd_out1/5(in_d04)
  pipeline136/1(q) -> cd_out1/4(in_d03)
  pipeline135/1(q) -> cd_out1/3(in_d02)
  pipeline134/1(q) -> cd_out1/2(in_d01)
  pipeline133/1(q) -> cd_out1/1(in_d00)
  bus_expand7/7(out2) -> pipeline139/1(d)
  bus_expand7/5(out4) -> pipeline137/1(d)
  bus_expand7/4(out5) -> pipeline136/1(d)
  bus_expand7/6(out3) -> pipeline138/1(d)
  bus_expand7/3(out6) -> pipeline135/1(d)
  bus_expand7/2(out7) -> pipeline134/1(d)
  pipeline142/1(q) -> cd_out1/9(in_dvalid)
  pipeline141/1(q) -> cd_out1/10(in_sync)
  pipeline147/1(q) -> cd_out1/12(trig)
  pipeline145/1(q) -> cd_out1/11(we)
  Logical13/1 -> pipeline145/1(d)
  [cd_dvalid] -> Logical13/1, pipeline142/1(d)
  bus_expand5/1(msb_out8) -> pipeline167/1(d)  "hmc_out9"
  bus_expand5/8(lsb_out1) -> pipeline76/1(d)  "hmc_out16"
  pipeline76/1(q) -> cd_out/8(in_d07)
  pipeline75/1(q) -> cd_out/7(in_d06)
  pipeline74/1(q) -> cd_out/6(in_d05)
  pipeline73/1(q) -> cd_out/5(in_d04)
  pipeline72/1(q) -> cd_out/4(in_d03)
  pipeline71/1(q) -> cd_out/3(in_d02)
  pipeline70/1(q) -> cd_out/2(in_d01)
  pipeline167/1(q) -> cd_out/1(in_d00)
  bus_expand5/7(out2) -> pipeline75/1(d)
  bus_expand5/5(out4) -> pipeline73/1(d)
  bus_expand5/4(out5) -> pipeline72/1(d)
  bus_expand5/6(out3) -> pipeline74/1(d)
  bus_expand5/3(out6) -> pipeline71/1(d)
  bus_expand5/2(out7) -> pipeline70/1(d)
  pipeline78/1(q) -> cd_out/9(in_dvalid)
  pipeline77/1(q) -> cd_out/10(in_sync)
  pipeline88/1(q) -> cd_out/12(trig)
  pipeline84/1(q) -> cd_out/11(we)
  Logical11/1 -> pipeline84/1(d)
  [cd_out_pol0] -> bus_expand4/1(bus_in), bus_expand5/1(bus_in)
  [cd_dvalid] -> pipeline78/1(d), Logical11/1
  cd_compensation0/2(dout) -> Gateway Out68/1, [cd_out_pol0]
  cd_compensation1/2(dout) -> Gateway Out69/1, [cd_out_pol1]
  cd_compensation0/1(sync_out) -> Gateway Out36/1, [cd_sync]
  cd_compensation0/3(dvalid) -> Gateway Out37/1, [cd_dvalid]
  hmc_error/1(sim_out) -> Terminator17/1
  [hmc_error] -> hmc_error/1(out_reg)
  hmc_parity_pol0/1(sim_out) -> Terminator14/1
  [hmc_parity_pol0] -> hmc_parity_pol0/1(out_reg)
  hmc_parity_pol1/1(sim_out) -> Terminator15/1
  [hmc_parity_pol1] -> hmc_parity_pol1/1(out_reg)
  cd_compensation0/4(hmc_error) -> [hmc_error]
  cd_compensation0/5(parity_error) -> [hmc_parity_pol0]
  cd_compensation1/5(parity_error) -> [hmc_parity_pol1]
  cd_compensation1/4(hmc_error) -> Terminator20/1
  cd_compensation1/3(dvalid) -> [cd_dvalid_pol1], Gateway Out67/1
  Constant24/1 -> [s256_d]
  Constant25/1 -> [s256_v]
  Constant26/1 -> [s256_eof]
  Constant2/1 -> [s256_of]
  Constant5/1 -> [s256_ip]
  Constant7/1 -> [s256_port]
  pipeline13/1(q) -> Gateway Out38/1, [tvg_adc_en]
  bus_expand4/1(msb_out8) -> Gateway Out/1
  bus_expand4/2(out7) -> Gateway Out1/1
  bus_expand4/3(out6) -> Gateway Out2/1
  bus_expand4/4(out5) -> Gateway Out3/1
  bus_expand4/5(out4) -> Gateway Out4/1
  bus_expand4/6(out3) -> Gateway Out5/1
  bus_expand4/7(out2) -> Gateway Out6/1
  bus_expand4/8(lsb_out1) -> Gateway Out7/1
  bus_expand8/8(lsb_out1) -> Gateway Out15/1
  bus_expand8/7(out2) -> Gateway Out14/1
  bus_expand8/6(out3) -> Gateway Out13/1
  bus_expand8/5(out4) -> Gateway Out12/1
  bus_expand8/4(out5) -> Gateway Out11/1
  bus_expand8/3(out6) -> Gateway Out10/1
  bus_expand8/2(out7) -> Gateway Out9/1
  bus_expand8/1(msb_out8) -> Gateway Out8/1
  Gateway Out7/1 -> To Workspace8/1
  Gateway Out6/1 -> To Workspace7/1
  Gateway Out5/1 -> To Workspace6/1
  Gateway Out4/1 -> To Workspace5/1
  Gateway Out3/1 -> To Workspace4/1
  Gateway Out2/1 -> To Workspace3/1
  Gateway Out1/1 -> To Workspace2/1
  Gateway Out/1 -> To Workspace/1
  Gateway Out8/1 -> To Workspace9/1
  Gateway Out9/1 -> To Workspace11/1
  Gateway Out10/1 -> To Workspace12/1
  Gateway Out11/1 -> To Workspace13/1
  Gateway Out12/1 -> To Workspace14/1
  Gateway Out13/1 -> To Workspace15/1
  Gateway Out14/1 -> To Workspace16/1
  Gateway Out15/1 -> To Workspace17/1
  Constant/1 -> [tvg_amp]
  Constant9/1 -> [tvg_offset]
  Gateway Out16/1 -> To Workspace1/1
  [tvg_offset] -> impulse0/1(sim_1)
  [tvg_amp] -> To Workspace10/1, impulse0/2(sim_2)
  [tvg_amp] -> impulse1/2(sim_2)
  [tvg_offset] -> impulse1/1(sim_1)
  bus_expand9/1(msb_out8) -> Gateway Out17/1
  bus_expand9/2(out7) -> Gateway Out18/1
  bus_expand9/3(out6) -> Gateway Out19/1
  bus_expand9/4(out5) -> Gateway Out20/1
  bus_expand9/5(out4) -> Gateway Out21/1
  bus_expand9/6(out3) -> Gateway Out22/1
  bus_expand9/7(out2) -> Gateway Out23/1
  bus_expand9/8(lsb_out1) -> Gateway Out24/1
  Gateway Out24/1 -> To Workspace26/1
  Gateway Out23/1 -> To Workspace25/1
  Gateway Out22/1 -> To Workspace24/1
  Gateway Out21/1 -> To Workspace23/1
  Gateway Out20/1 -> To Workspace22/1
  Gateway Out19/1 -> To Workspace21/1
  Gateway Out18/1 -> To Workspace20/1
  Gateway Out17/1 -> To Workspace18/1
  [d80_adc0] -> bus_expand9/1(bus_in)
  bus_expand10/1(msb_out8) -> Gateway Out25/1
  bus_expand10/2(out7) -> Gateway Out26/1
  bus_expand10/3(out6) -> Gateway Out27/1
  bus_expand10/4(out5) -> Gateway Out28/1
  bus_expand10/5(out4) -> Gateway Out29/1
  bus_expand10/6(out3) -> Gateway Out30/1
  bus_expand10/7(out2) -> Gateway Out31/1
  bus_expand10/8(lsb_out1) -> Gateway Out32/1
  Gateway Out32/1 -> To Workspace34/1
  Gateway Out31/1 -> To Workspace33/1
  Gateway Out30/1 -> To Workspace32/1
  Gateway Out29/1 -> To Workspace31/1
  Gateway Out28/1 -> To Workspace30/1
  Gateway Out27/1 -> To Workspace29/1
  Gateway Out26/1 -> To Workspace28/1
  Gateway Out25/1 -> To Workspace19/1
  [d80_adc1] -> bus_expand10/1(bus_in)
  Gateway Out33/1 -> To Workspace27/1
  Gateway Out34/1 -> To Workspace35/1
  Gateway Out35/1 -> To Workspace36/1
  Gateway Out36/1 -> To Workspace37/1
  Gateway Out37/1 -> To Workspace38/1
  Constant8/1 -> control/1(sim_1)
  Constant11/1 -> control/2(sim_2)
  Constant14/1 -> control/3(sim_3)
  Constant15/1 -> control/4(sim_4)
  Constant18/1 -> control/5(sim_5)
  Constant19/1 -> control/6(sim_6)
  Constant20/1 -> control/7(sim_7)
  Constant21/1 -> control/8(sim_8)
  Constant22/1 -> control/9(sim_9)
  Constant23/1 -> control/10(sim_10)
  Gateway Out38/1 -> To Workspace39/1
  Gateway Out39/1 -> To Workspace40/1
  Gateway Out40/1 -> To Workspace41/1
  pipeline2/1(q) -> db_trig/1(out_reg)
  Counter1/1 -> pipeline2/1(d)
  [sys_rst] -> Counter1/1
  pipeline4/1(q) -> db_dvalid/1(out_reg)
  Counter2/1 -> pipeline4/1(d)
  [sys_rst] -> Counter3/1, Counter5/1, Counter4/1, Counter2/1
  pipeline8/1(q) -> db_sync/1(out_reg)
  Counter3/1 -> pipeline8/1(d)
  pipeline9/1(q) -> db_unpack_dvalid/1(out_reg)
  Counter4/1 -> pipeline9/1(d)
  [sync80] -> Counter3/2
  [unpack_dv] -> Counter4/2
  pipeline27/1(q) -> db_unpack_sync/1(out_reg)
  Counter5/1 -> pipeline27/1(d)
  [unpack_sync] -> Counter5/2
  [cd_out_ss_trig_pol0] -> pipeline77/1(d), Logical11/2, pipeline88/1(d)
  pipeline29/1(q) -> cd_out1/13(stop)
  pipeline30/1(q) -> cd_out/13(stop)
  count_rst/1(in_rst) -> edge_detect20/1(in)
  Counter15/1 -> Relational/1, Gateway Out48/1
  Relational/1 -> edge_detect23/1(in), Gateway Out43/1
  Constant27/1 -> Relational/2
  [count_rst] -> Counter17/1
  Register16/1 -> [cd_out_ss_stop_pol0], Inverter11/1
  Logical31/1 -> Gateway Out59/1, Logical33/2
  Inverter11/1 -> Gateway Out58/1, Logical31/1
  Counter17/1 -> cd_data_pol0_delay/1(out_reg)
  cd_data_pol0_delay/1(sim_out) -> To Workspace65/1
  edge_detect24/1(out) -> Gateway Out61/1, Register16/3, Register16/1, Counter19/2
  Counter19/1 -> cd_out_pol0_count/1(out_reg)
  cd_out_pol0_count/1(sim_out) -> To Workspace67/1
  Logical33/1 -> Gateway Out47/1, Counter17/2
  [cd_dvalid] -> Logical33/1
  Impulse_detect5/1(Out1) -> Gateway Out42/1, edge_detect24/1(in)
  Gateway Out41/1 -> To Workspace61/1
  Gateway Out42/1 -> To Workspace62/1
  Gateway Out43/1 -> To Workspace63/1
  Gateway Out47/1 -> To Workspace70/1
  Gateway Out48/1 -> To Workspace71/1
  Gateway Out58/1 -> To Workspace84/1
  Gateway Out59/1 -> To Workspace85/1
  [cd_out_pol0] -> Delay5/1
  Gateway Out61/1 -> To Workspace87/1
  Logical32/1 -> Relational/3, Gateway Out44/1, Counter15/2
  [sys_rst] -> Counter15/1, Gateway Out41/1, Register17/2
  Gateway Out44/1 -> To Workspace64/1
  edge_detect23/1(out) -> Register15/3, Register15/1, Gateway Out46/1
  Register15/1 -> Gateway Out45/1, Logical31/2, [cd_out_ss_trig_pol0]
  Gateway Out45/1 -> To Workspace68/1
  Gateway Out46/1 -> To Workspace69/1
  Constant29/1 -> delay1/1(sim_1), delay0/1(sim_1)
  edge_detect20/1(out) -> [count_rst]
  [count_rst] -> Register15/2
  [count_rst] -> Counter19/1, Register16/2
  Counter14/1 -> Gateway Out56/1, Relational1/1
  Relational1/1 -> Gateway Out51/1, edge_detect21/1(in)
  Constant13/1 -> Relational1/2
  [count_rst] -> Counter16/1
  Register19/1 -> Inverter12/1
  Logical24/1 -> Logical35/2, Gateway Out60/1
  Inverter12/1 -> Logical24/1, Gateway Out57/1
  Counter16/1 -> d80_data_delay/1(out_reg)
  d80_data_delay/1(sim_out) -> To Workspace75/1
  edge_detect22/1(out) -> Counter21/2, Register19/1, Register19/3, Gateway Out62/1
  Counter20/1 -> spec_edge_count/1(out_reg)
  spec_edge_count/1(sim_out) -> To Workspace76/1
  Counter21/1 -> d80_pol0_count/1(out_reg)
  d80_pol0_count/1(sim_out) -> To Workspace77/1
  Logical35/1 -> Counter16/2, Gateway Out55/1
  [valid80] -> Logical35/1
  Impulse_detect6/1(Out1) -> edge_detect22/1(in), Gateway Out50/1
  Gateway Out49/1 -> To Workspace60/1
  Gateway Out50/1 -> To Workspace72/1
  Gateway Out51/1 -> To Workspace73/1
  Gateway Out55/1 -> To Workspace80/1
  Gateway Out56/1 -> To Workspace81/1
  Gateway Out57/1 -> To Workspace82/1
  Gateway Out60/1 -> To Workspace83/1
  Delay9/1 -> Impulse_detect6/1(In1)
  Gateway Out62/1 -> To Workspace86/1
  Logical34/1 -> Counter14/2, Gateway Out52/1, Relational1/3
  [valid80] -> Delay4/1
  Register20/1 -> Logical34/2
  [sys_rst] -> Register20/2, Gateway Out49/1, Counter14/1
  [sync80] -> Register20/1, Register20/3
  [d80_adc0] -> Delay9/1
  Gateway Out52/1 -> To Workspace74/1
  edge_detect21/1(out) -> Gateway Out54/1, Register18/1, Counter20/2, Register18/3
  Register18/1 -> Logical24/2, Gateway Out53/1
  Gateway Out53/1 -> To Workspace78/1
  Gateway Out54/1 -> To Workspace79/1
  [count_rst] -> Register18/2, Counter20/1
  [count_rst] -> Register19/2, Counter21/1
  Counter6/1 -> Relational2/1
  Relational2/1 -> edge_detect3/1(in)
  Constant28/1 -> Relational2/2
  [count_rst] -> Counter7/1
  Register2/1 -> [cd_out_ss_stop_pol1], Inverter3/1
  Logical4/1 -> Logical9/2
  Inverter3/1 -> Logical4/1
  Counter7/1 -> cd_data_pol1_delay/1(out_reg)
  cd_data_pol1_delay/1(sim_out) -> To Workspace46/1
  edge_detect5/1(out) -> Counter8/2, Register2/1, Register2/3
  Counter8/1 -> cd_out_pol1_count/1(out_reg)
  cd_out_pol1_count/1(sim_out) -> To Workspace47/1
  Logical9/1 -> Counter7/2
  [cd_dvalid_pol1] -> Logical9/1
  Impulse_detect1/1(Out1) -> edge_detect5/1(in)
  [cd_out_pol1] -> Delay6/1
  Logical8/1 -> Counter6/2, Relational2/3
  Register3/1 -> Logical8/2
  [sys_rst] -> Register3/2, Counter6/1
  [cd_sync_pol1] -> Register3/1, Register3/3
  edge_detect3/1(out) -> Register1/1, Register1/3
  Register1/1 -> [cd_out_ss_trig_pol1], Logical4/2
  [count_rst] -> Register1/2
  [count_rst] -> Register2/2, Counter8/1
  [cd_dvalid_pol1] -> Logical8/1
  [cd_dvalid] -> Logical32/1
  Delay4/1 -> Logical34/1
  [cd_out_ss_stop_pol0] -> pipeline30/1(d)
  [cd_out_ss_trig_pol1] -> pipeline141/1(d), Logical13/2, pipeline147/1(d)
  [cd_out_ss_stop_pol1] -> pipeline29/1(d)
  Gateway Out63/1 -> To Workspace42/1
  Gateway Out64/1 -> To Workspace43/1
  Gateway Out65/1 -> To Workspace44/1
  Gateway Out66/1 -> To Workspace45/1
  Gateway Out67/1 -> To Workspace48/1
  Gateway Out68/1 -> To Workspace49/1
  Gateway Out69/1 -> To Workspace50/1
  Gateway Out175/1 -> To Workspace201/1
  Gateway Out70/1 -> To Workspace51/1
  Gateway Out71/1 -> To Workspace52/1
  Register17/1 -> Gateway Out71/1, Logical32/2
  Delay5/1 -> Impulse_detect5/1(In1)
  Delay6/1 -> Impulse_detect1/1(In1)
  [unpack_dv] -> Gateway Out40/1, sync_gen/2(en)
  Constant10/1 -> Terminator3/1
  [cd_sync] -> Register17/3, Register17/1
  cd_compensation1/1(sync_out) -> [cd_sync_pol1], Gateway Out66/1
